simulink model "double_line_system"  (R2018a)
settings: Solver=ode45  StartTime=0.0  StopTime=4/60  FixedStep=Ts  RelTol=1e-3
PreLoadFcn:
  | gr
libraries: powerlib x10
(part 2 of 2)

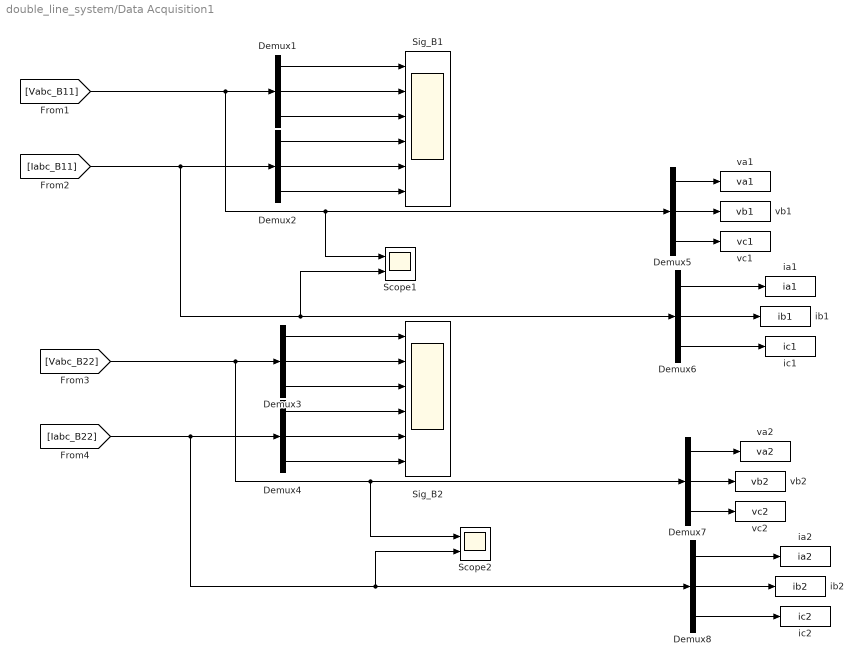
== system double_line_system/Data Acquisition1 ==
  Demux{1..8} (8 alike) : Demux  Outputs=3
  Scope1 : Scope  NumInputPorts=2
  Scope2 : Scope  NumInputPorts=2
  Sig_B1 : Scope  NumInputPorts=6
  Sig_B2 : Scope  NumInputPorts=6
  ia1 : ToWorkspace  VariableName=ia1  SampleTime=1/2160
  ia2 : ToWorkspace  VariableName=ia2  SampleTime=1/2160
  ib1 : ToWorkspace  VariableName=ib1  SampleTime=1/2160
  ib2 : ToWorkspace  VariableName=ib2  SampleTime=1/2160
  ic1 : ToWorkspace  VariableName=ic1  SampleTime=1/2160
  ic2 : ToWorkspace  VariableName=ic2  SampleTime=1/2160
  va1 : ToWorkspace  VariableName=va1  SampleTime=1/2160
      settings: MaxDataPoints=5000000
  va2 : ToWorkspace  VariableName=va2  SampleTime=1/2160
  vb1 : ToWorkspace  VariableName=vb1  SampleTime=1/2160
      settings: MaxDataPoints=5000000
  vb2 : ToWorkspace  VariableName=vb2  SampleTime=1/2160
  vc1 : ToWorkspace  VariableName=vc1  SampleTime=1/2160
      settings: MaxDataPoints=5000000
  vc2 : ToWorkspace  VariableName=vc2  SampleTime=1/2160
  wires:
  Demux1/1 -> Sig_B1/1
  Demux1/2 -> Sig_B1/2
  Demux1/3 -> Sig_B1/3
  Demux2/1 -> Sig_B1/4
  Demux2/2 -> Sig_B1/5
  Demux2/3 -> Sig_B1/6
  Demux3/1 -> Sig_B2/1
  Demux3/2 -> Sig_B2/2
  Demux3/3 -> Sig_B2/3
  Demux4/1 -> Sig_B2/4
  Demux4/2 -> Sig_B2/5
  Demux4/3 -> Sig_B2/6
  [Vabc_B11] -> Demux1/1, Demux5/1, Scope1/1
  [Iabc_B11] -> Demux2/1, Demux6/1, Scope1/2
  [Vabc_B22] -> Demux3/1, Demux7/1, Scope2/1
  [Iabc_B22] -> Demux4/1, Demux8/1, Scope2/2
  Demux5/1 -> va1/1
  Demux5/2 -> vb1/1
  Demux5/3 -> vc1/1
  Demux6/1 -> ia1/1
  Demux6/2 -> ib1/1
  Demux6/3 -> ic1/1
  Demux7/1 -> va2/1
  Demux7/2 -> vb2/1
  Demux7/3 -> vc2/1
  Demux8/1 -> ia2/1
  Demux8/2 -> ib2/1
  Demux8/3 -> ic2/1
